simulink model "ParallelServerModel"  (R2025a)
settings: Solver=VariableStepAuto  StartTime=0.0  StopTime=10.0  RelTol=1e-3
values from neighbouring files (symbols this model uses):
  K = 5    [main.m]
  lambda = lambda_values(i)    [main.m]
  mu = 1.0    (= 1)    [main.m]
  Tstop = 100    [main.m]
settings Model: Creator=asssf  LastModifiedBy=asssf

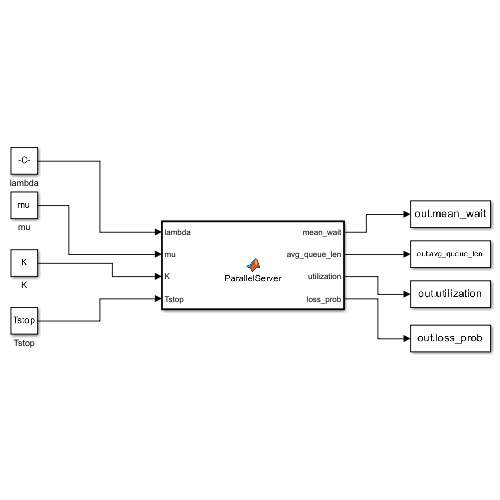
[thumbnail: Simulink's stored preview of the top-level diagram]
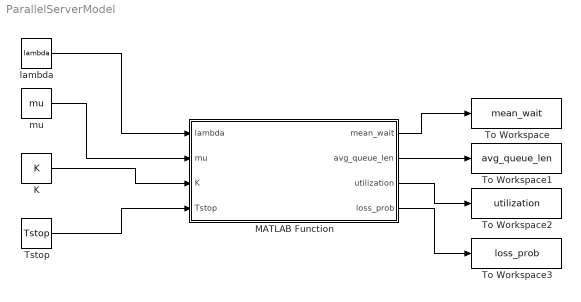
== system ParallelServerModel ==
  K : Constant  Value=K
  MATLAB Function : MATLAB Function  TreatAsAtomicUnit=on
  To Workspace : ToWorkspace  VariableName=mean_wait  SaveFormat=Timeseries  SampleTime=-1
  To Workspace1 : ToWorkspace  VariableName=avg_queue_len  SaveFormat=Timeseries  SampleTime=-1
  To Workspace2 : ToWorkspace  VariableName=utilization  SaveFormat=Timeseries  SampleTime=-1
  To Workspace3 : ToWorkspace  VariableName=loss_prob  SaveFormat=Timeseries  SampleTime=-1
  Tstop : Constant  Value=Tstop
  lambda : Constant  Value=lambda
  mu : Constant  Value=mu
  wires:
  lambda/1 -> MATLAB Function/1(lambda)
  mu/1 -> MATLAB Function/2(mu)
  K/1 -> MATLAB Function/3(K)
  Tstop/1 -> MATLAB Function/4(Tstop)
  MATLAB Function/1(mean_wait) -> To Workspace/1
  MATLAB Function/2(avg_queue_len) -> To Workspace1/1
  MATLAB Function/3(utilization) -> To Workspace2/1
  MATLAB Function/4(loss_prob) -> To Workspace3/1

== matlab function ParallelServerModel/MATLAB Function ==
  data: lambda input; mean_wait output; mu input; K input; Tstop input; avg_queue_len output; utilization output; loss_prob output
function [mean_wait, avg_queue_len, utilization, loss_prob] = ParallelServer(lambda, mu, K, Tstop)
% --- Вхідні параметри ---
lambda = double(lambda);
mu = double(mu);
K = double(K);
Tstop = double(Tstop);

% Якщо розмір черги K не вказано (<=0), вважаємо її нескінченною
if K <= 0
    K = Inf;
end

% --- Ініціалізація симуляції ---
nservers = 2;          % Кількість серверів
t = 0;                 % Поточний час симуляції

% Планування першої заявки
if lambda > 0
    t_arr = -log(rand)/lambda;
else
    t_arr = Inf;
end

% Ініціалізація стану серверів та черги
service_end = Inf(1, nservers);  
busy = zeros(1, nservers);
queue = [];              

% Ініціалізація статистики
area_q = 0;               
area_busy = 0;            
arrivals = 0;
losses = 0;
served = 0;
sum_wait = 0;

% --- Головний цикл симуляції ---
while t < Tstop
   
    t_service_min = min(service_end);
    
    % --- Випадок 1: Наступна подія - прибуття заявки ---
    if t_arr <= t_service_min
        
        tnext = t_arr;
        if tnext > Tstop
            break;
        end
        
        % Оновлення статистики на інтервалі [t, tnext]
        dt = tnext - t;
        area_q = area_q + numel(queue)*dt;
        area_busy = area_busy + sum(busy)*dt;
        
        t = tnext;
        arrivals = arrivals + 1;
       
        % Пошук вільного сервера
        free_idx = find(busy==0, 1);
        if ~isempty(free_idx) % Якщо є вільний сервер
            busy(free_idx) = 1;
            service_time = -log(rand)/mu;
            service_end(free_idx) = t + service_time;
        else % Якщо всі сервери зайняті
            if numel(queue) >= K
                losses = losses + 1; % Заявка втрачається
            else
                queue(end+1) = t; % Заявка стає в чергу
            end
        end
      
        % Планування наступної заявки
        if lambda > 0
            t_arr = t + (-log(rand)/lambda);
        else
            t_arr = Inf;
        end
        
    % --- Випадок 2: Наступна подія - завершення обслуговування ---
    else
        tnext = t_service_min;
        if tnext > Tstop
            break;
        end
        
        % Оновлення статистики
        dt = tnext - t;
        area_q = area_q + numel(queue)*dt;
        area_busy = area_busy + sum(busy)*dt;
        t = tnext;
        
        % Знаходимо, які саме сервери звільнилися
        idx = find(abs(service_end - t) < 1e-12);
        
        % --- ВИПРАВЛЕНО ---
        % Цикл, який розуміє Simulink Coder
        for i = 1:numel(idx)
            j = idx(i);
            
            if ~isempty(queue) % Якщо черга не порожня
                arrival_time = queue(1);
                queue(1) = []; % Видаляємо заявку з черги
                
                wait = t - arrival_time;
                sum_wait = sum_wait + wait;
                served = served + 1;
                
                % Відразу починаємо обслуговувати нову заявку
                service_time = -log(rand)/mu;
                service_end(j) = t + service_time;
                busy(j) = 1; % Сервер залишається зайнятим
            else % Якщо черга порожня
                busy(j) = 0; % Сервер стає вільним
                service_end(j) = Inf;
            end
        end
    end
end

% --- Розрахунок фінальних показників ---
if served > 0
    mean_wait = sum_wait / served;
else
    mean_wait = 0;
end

avg_queue_len = area_q / Tstop;
utilization = area_busy / (nservers * Tstop);

if arrivals > 0
    loss_prob = losses / arrivals;
else
    loss_prob = 0;
end

end
